simulink model "orbit_validation_init"  (Simulink 6.2)
settings: Solver=FixedStepDiscrete  StartTime=0.0  StopTime=10000  RelTol=1e-3
libraries: components_lib x3, ephemeris_lib x1, simulink_extras x1
settings Model: LastModifiedBy=rals  ExtModeAutoUpdateStatusClock=off
settings DebuggingCC: SolverPrmCheckMsg=warning

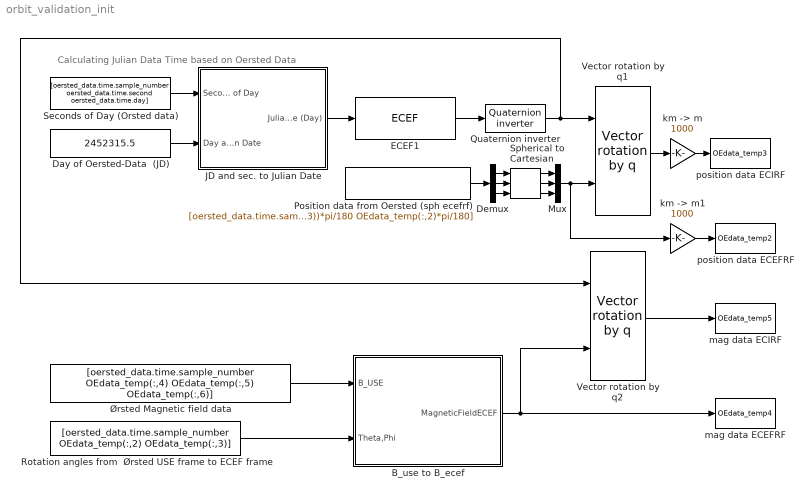
== system orbit_validation_init ==
  note: Calculating Julian Data Time based on Oersted Data
  B_use to B_ecef : Subsystem
  Day of Oersted-Data  (JD) : Constant  Value=2452315.5
  Demux : Demux  Outputs=3
  ECEF1 : ephemeris_lib/Ephemeris/ECEF
  JD and sec. to Julian Date : Subsystem
  Mux : Mux  Inputs=3
  Position data from Oersted (sph ecefrf) : FromWorkspace  VariableName=[oersted_data.time.sample_number OEdata_temp(:,1) (OEdata_temp(:,3))*pi/180 OEdata_temp(:,2)*pi/180]  SampleTime=1
  Quaternion inverter : components_lib/Math utilities/Quaternion operations/Quaternion inverter
  Rotation angles from  Ørsted USE frame to ECEF frame : FromWorkspace  VariableName=[oersted_data.time.sample_number OEdata_temp(:,2) OEdata_temp(:,3)]  SampleTime=1
  Seconds of Day (Orsted data) : FromWorkspace  VariableName=[oersted_data.time.sample_number oersted_data.time.second oersted_data.time.day]  SampleTime=1
  Spherical to Cartesian : simulink_extras/Transformations/Spherical to Cartesian
  Vector rotation by q1 : components_lib/Math utilities/Vector operations/Vector rotation by q
  Vector rotation by q2 : components_lib/Math utilities/Vector operations/Vector rotation by q
  "km -> m" : Gain  Gain=1000  SaturateOnIntegerOverflow=on
  "km -> m1" : Gain  Gain=1000  SaturateOnIntegerOverflow=on
  mag data ECEFRF : ToWorkspace  VariableName=OEdata_temp4  SampleTime=-1  SaveFormat=Array
  mag data ECIRF : ToWorkspace  VariableName=OEdata_temp5  SampleTime=-1  SaveFormat=Array
  position data ECEFRF : ToWorkspace  VariableName=OEdata_temp2  SampleTime=-1  SaveFormat=Array
  position data ECIRF : ToWorkspace  VariableName=OEdata_temp3  SampleTime=-1  SaveFormat=Array
  "Ørsted Magnetic field data " : FromWorkspace  VariableName=[oersted_data.time.sample_number OEdata_temp(:,4) OEdata_temp(:,5) OEdata_temp(:,6)]  SampleTime=1
  wires:
  Seconds of Day (Orsted data)/1 -> JD and sec. to Julian Date/1(Second of Day)
  Vector rotation by q1/1 -> "km -> m"/1
  Day of Oersted-Data  (JD)/1 -> JD and sec. to Julian Date/2(Day as Julian Date)
  Quaternion inverter/1 -> Vector rotation by q1/1, Vector rotation by q2/1
  JD and sec. to Julian Date/1(Julian Date (Day)) -> ECEF1/1
  ECEF1/1 -> Quaternion inverter/1
  "Ørsted Magnetic field data "/1 -> B_use to B_ecef/1(B_USE)
  Rotation angles from  Ørsted USE frame to ECEF frame/1 -> B_use to B_ecef/2(Theta,Phi)
  B_use to B_ecef/1(MagneticFieldECEF) -> mag data ECEFRF/1, Vector rotation by q2/2
  Vector rotation by q2/1 -> mag data ECIRF/1
  Demux/1 -> Spherical to Cartesian/1
  Position data from Oersted (sph ecefrf)/1 -> Demux/1
  Demux/3 -> Spherical to Cartesian/3
  Demux/2 -> Spherical to Cartesian/2
  Spherical to Cartesian/1 -> Mux/1
  Spherical to Cartesian/2 -> Mux/2
  Spherical to Cartesian/3 -> Mux/3
  Mux/1 -> Vector rotation by q1/2, "km -> m1"/1
  "km -> m"/1 -> position data ECIRF/1
  "km -> m1"/1 -> position data ECEFRF/1

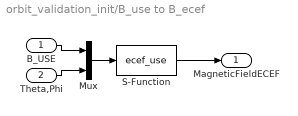
== system orbit_validation_init/B_use to B_ecef ==
  B_USE : Inport  Port=1  LatchInput=off
  Theta,Phi : Inport  Port=2  LatchInput=off
  Mux : Mux  Inputs=2
  S-Function : S-Function  FunctionName=ecef_use
  MagneticFieldECEF : Outport
  wires:
  B_USE/1 -> Mux/1
  Theta,Phi/1 -> Mux/2
  Mux/1 -> S-Function/1
  S-Function/1 -> MagneticFieldECEF/1

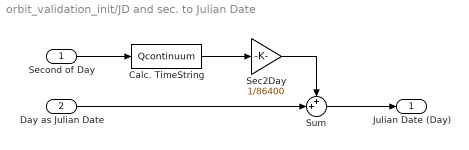
== system orbit_validation_init/JD and sec. to Julian Date ==
  Second of Day : Inport  Port=1  LatchInput=off
  Day as Julian Date : Inport  Port=2  LatchInput=off
  Calc. TimeString : S-Function  FunctionName=Qcontinuum
  Sec2Day : Gain  Gain=1/86400  SaturateOnIntegerOverflow=on
  Sum : Sum  Inputs=++|  SaturateOnIntegerOverflow=on  InputSameDT=on
  Julian Date (Day) : Outport
  wires:
  Sum/1 -> Julian Date (Day)/1
  Second of Day/1 -> Calc. TimeString/1
  Day as Julian Date/1 -> Sum/2
  Sec2Day/1 -> Sum/1
  Calc. TimeString/1 -> Sec2Day/1
